simulink model "Current_Sensor_INA219"  (R2022a)
settings: Solver=VariableStepAuto  StartTime=0.0  StopTime=10.0  RelTol=1e-3
libraries: arduinolib x4
settings Model: Creator=sokse  LastModifiedBy=sokse

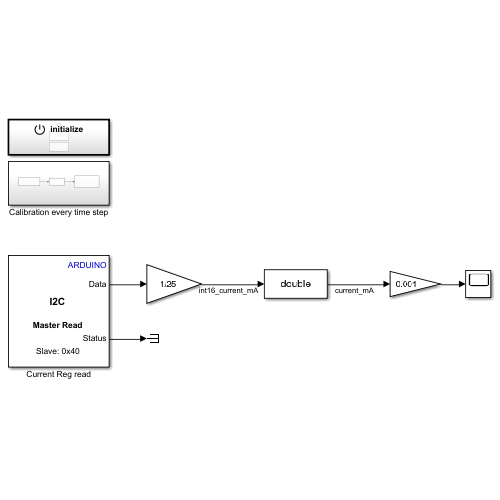
[thumbnail: Simulink's stored preview of the top-level diagram]
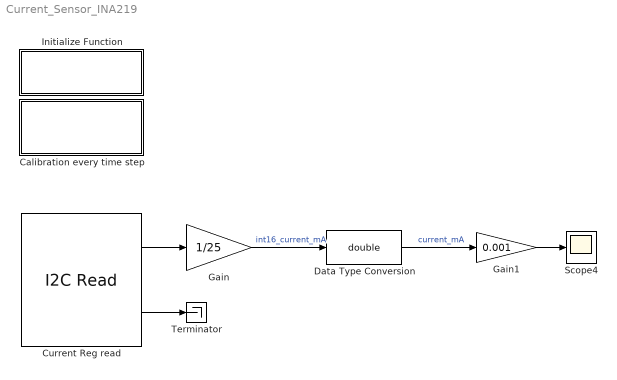
== system Current_Sensor_INA219 ==
  Calibration every time step : Subsystem  Priority=0
  Current Reg read : arduinolib/I2C Read  I2CModule=0  Mode=Master  SlaveAddress="hex2dec(\"0x40\")"  SlaveByteOrder=BigEndian  Direction=Receiver  RegisterAddressMode=on  RegisterAddress="hex2dec(\"0x04\")"  SlaveDataType=int16  DataLength=1  NoAck=off  RepeatedStart=off  OutputStatus=on  blockPlatform=ARDUINO  SampleTime=0.1
      settings: SourceProductBaseCode=ARDUINO
  Data Type Conversion : DataTypeConversion  OutDataTypeStr=double  SaturateOnIntegerOverflow=off  RndMeth=Floor
  Gain : Gain  Gain=1/25
  Gain1 : Gain  Gain=0.001
  Initialize Function : Subsystem  TreatAsAtomicUnit=on
  Scope4 : Scope
  Terminator : Terminator
  wires:
  Data Type Conversion/1 -> Gain1/1  "current_mA"
  Current Reg read/2 -> Terminator/1
  Current Reg read/1 -> Gain/1
  Gain/1 -> Data Type Conversion/1  "int16_current_mA"
  Gain1/1 -> Scope4/1

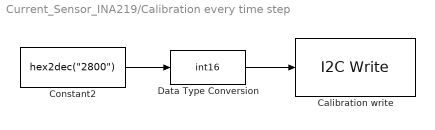
== system Current_Sensor_INA219/Calibration every time step ==
  Calibration write : arduinolib/I2C Write  I2CModule=0  Mode=Master  SlaveAddress="uint8(hex2dec(\"0x40\"))"  SlaveByteOrder=BigEndian  Direction=Transmitter  RegisterAddressMode=on  RegisterAddress="uint8(hex2dec(\"0x05\"))"  SlaveDataType=uint8  DataLength=1  NoAck=off  RepeatedStart=off  OutputStatus=off  blockPlatform=ARDUINO
      settings: SourceProductBaseCode=ARDUINO
  Constant2 : Constant  Value="hex2dec(\"2800\")"
  Data Type Conversion : DataTypeConversion  OutDataTypeStr=int16  SaturateOnIntegerOverflow=off  RndMeth=Floor
  wires:
  Constant2/1 -> Data Type Conversion/1
  Data Type Conversion/1 -> Calibration write/1

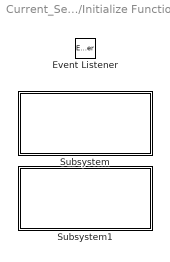
== system Current_Sensor_INA219/Initialize Function ==
  Event Listener : EventListener  DisableCoverage=on  EventName=reset
  Subsystem : Subsystem  Priority=0
  Subsystem1 : Subsystem  Priority=1

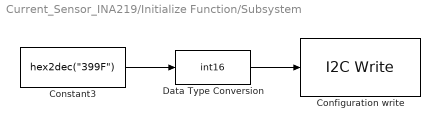
== system Current_Sensor_INA219/Initialize Function/Subsystem ==
  Configuration write : arduinolib/I2C Write  I2CModule=0  Mode=Master  SlaveAddress="hex2dec(\"0x40\")"  SlaveByteOrder=BigEndian  Direction=Transmitter  RegisterAddressMode=on  RegisterAddress="hex2dec(\"0x00\")"  SlaveDataType=uint8  DataLength=1  NoAck=off  RepeatedStart=off  OutputStatus=off  blockPlatform=ARDUINO
      settings: SourceProductBaseCode=ARDUINO
  Constant3 : Constant  Value="hex2dec(\"399F\")"
  Data Type Conversion : DataTypeConversion  OutDataTypeStr=int16  SaturateOnIntegerOverflow=off  RndMeth=Floor
  wires:
  Constant3/1 -> Data Type Conversion/1
  Data Type Conversion/1 -> Configuration write/1

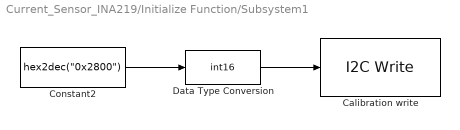
== system Current_Sensor_INA219/Initialize Function/Subsystem1 ==
  Calibration write : arduinolib/I2C Write  I2CModule=0  Mode=Master  SlaveAddress="uint8(hex2dec(\"0x40\"))"  SlaveByteOrder=BigEndian  Direction=Transmitter  RegisterAddressMode=on  RegisterAddress="uint8(hex2dec(\"0x05\"))"  SlaveDataType=uint8  DataLength=1  NoAck=off  RepeatedStart=off  OutputStatus=off  blockPlatform=ARDUINO
      settings: SourceProductBaseCode=ARDUINO
  Constant2 : Constant  Value="hex2dec(\"0x2800\")"
  Data Type Conversion : DataTypeConversion  OutDataTypeStr=int16  SaturateOnIntegerOverflow=off  RndMeth=Floor
  wires:
  Constant2/1 -> Data Type Conversion/1
  Data Type Conversion/1 -> Calibration write/1
